simulink subsystem "convert_32_16_to_8"  (R2022b)
settings: Solver=VariableStepAuto  StartTime=0.0  StopTime=10.0  RelTol=1e-3
settings Model: Creator=Ali-Laptop  LastModifiedBy=Ali-Laptop

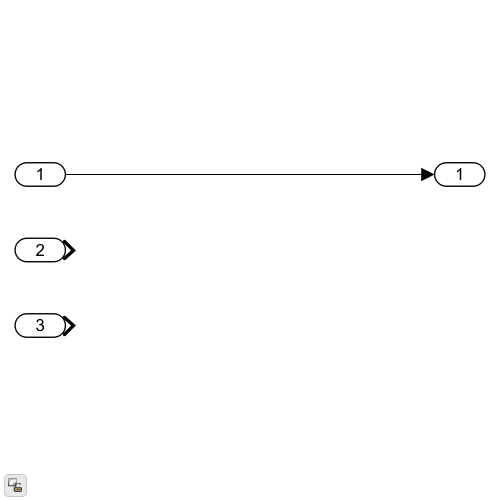
[thumbnail: Simulink's stored preview of the top-level diagram]
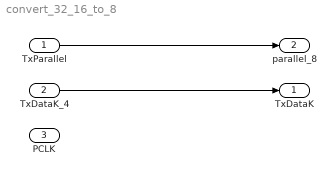
== system convert_32_16_to_8 ==
  TxParallel : Inport
  TxDataK_4 : Inport  Port=2
  PCLK : Inport  Port=3
  TxDataK : Outport
  parallel_8 : Outport  Port=2
  wires:
  TxDataK_4/1 -> TxDataK/1
  TxParallel/1 -> parallel_8/1
